simulink model "TestNozzleUnchoked"  (R2013b)
settings: Solver=ode45  StartTime=0.0  StopTime=10.0  RelTol=1e-3
libraries: Lib_TurboC_FlowStart_TMATSC x1, Lib_TurboC_Nozzle_TMATSC x1
settings Model: Creator=tlavelle  LastModifiedBy=jwchapm2
settings OptimizationCC: ExpressionDepthLimit=2147483647
settings DebuggingCC: StateNameClashWarn=warning

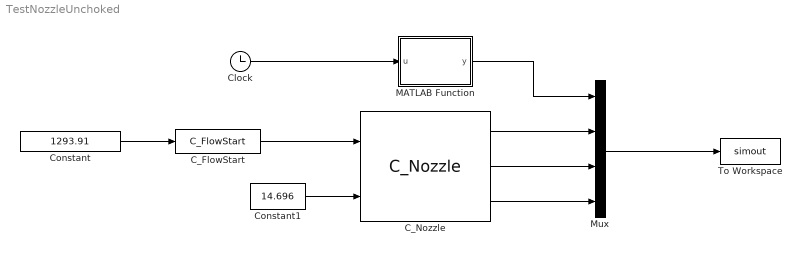
== system TestNozzleUnchoked ==
  C_FlowStart : Lib_TurboC_FlowStart_TMATSC/C_FlowStart  Tt_M=632.71  Pt_M=23.195  comp1_M=1  comp2_M=0  comp3_M=0  comp4_M=0  comp5_M=0  comp6_M=0
  C_Nozzle : Lib_TurboC_Nozzle_TMATSC/C_Nozzle  Ath_in_M=2706.36  Cfg_M=.9975  IDes_M=2  Wdes_M=1293
  Clock : Clock
  Constant : Constant  Value=1293.91
  Constant1 : Constant  Value=14.696
  MATLAB Function : MATLAB Function  TreatAsAtomicUnit=on
  Mux : Mux
  To Workspace : ToWorkspace  VariableName=simout  SampleTime=-1  SaveFormat=Timeseries
  wires:
  Constant/1 -> C_FlowStart/1
  C_FlowStart/1 -> C_Nozzle/1
  Constant1/1 -> C_Nozzle/2
  Clock/1 -> MATLAB Function/1(u)
  Mux/1 -> To Workspace/1
  C_Nozzle/1 -> Mux/2
  C_Nozzle/2 -> Mux/3
  C_Nozzle/3 -> Mux/4
  MATLAB Function/1(y) -> Mux/1

== matlab function TestNozzleUnchoked/MATLAB Function ==
  data: u input; y output
function y = fcn(u)
%#codegen
eml.extrinsic('set_param');
if u < 3
   set_param('TestNozzleUnChoked/C_Nozzle','IDes_M','0');
elseif u< 6 
   set_param('TestNozzleUnChoked/C_Nozzle','IDes_M','1'); 
else 
   set_param('TestNozzleUnChoked/C_Nozzle','IDes_M','2'); 
end    
y = u;
